simulink model "BOoe221SystReel"  (R2017a)
settings: Solver=VariableStepAuto  StartTime=0.0  StopTime=1000  RelTol=1e-9
values from neighbouring files (symbols this model uses):
  Ac75 = [26.3183614036 4.0966592869 -1.20233311116 0.735865601479 -0.745822636963 1.2499757532 -4.34795583254 -48.1646836676 11.3086114423 8.50188757288 -3.89847108842 3.46848516105 ... (49 elements, 7x7)]    [robot_75.mat]
  B = oe221.B    [main.m]
  Bc75 = [3.2987807581 -0.797878528803 0.404454582357 -0.331411019122 0.414411617841 -0.835564135359 3.51239169718]    [robot_75.mat]
  Cc75 = [0.0368 0.0059 -0.1248 0.3042 -0.2181 0.0895 0]    [robot_75.mat]
  F = oe221.F    [main.m]
  Te = 0.07    [robot_0.mat]    (also in robot_25.mat; robot_75.mat)
undefined symbols (not defined in the file or in its folder): DiscIntNeverNeededParam
libraries: simulink x2
settings Model: Creator=GANOU Arouna  LastModifiedBy=GANOU Arouna

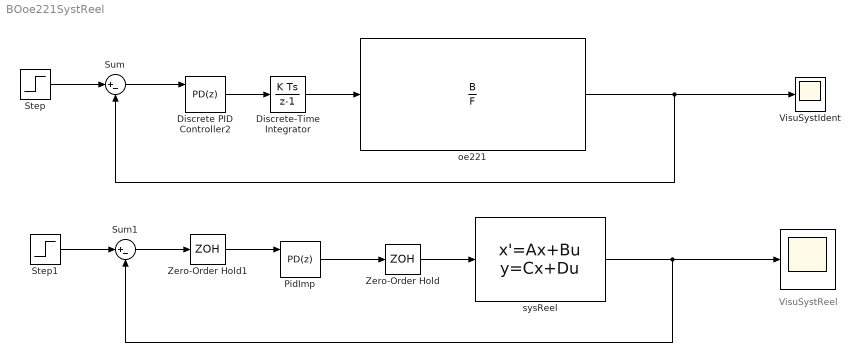
== system BOoe221SystReel ==
  note: VisuSystReel
  " " : Scope
  Discrete PID Controller2 : simulink/Continuous/PID Controller  Controller=PD  TimeDomain=Discrete-time  SampleTime=Te  IntegratorMethod=Forward Euler  FilterMethod=Forward Euler  Form=Parallel  UseFilter=on  ControllerParametersSource=internal  P=0.00429057698105191  I=0.0008007758385471  D=0  N=100  InitialConditionSource=internal  InitialConditionForIntegrator=0  InitialConditionForFilter=0  ExternalReset=either  LimitOutput=off  UpperSaturationLimit=inf  LowerSaturationLimit=-inf  LinearizeAsGain=off  AntiWindupMode=none  Kb=1  TrackingMode=off  Kt=1  PParamMin=[]  PParamMax=[]  IParamMin=[]  IParamMax=[]  DParamMin=[]  DParamMax=[]  NParamMin=[]  NParamMax=[]  KbParamMin=[]  KbParamMax=[]  KtParamMin=[]  KtParamMax=[]  POutMin=[]  POutMax=[]  IOutMin=[]  IOutMax=[]  DOutMin=[]  DOutMax=[]  NOutMin=[]  NOutMax=[]  KbOutMin=[]  KbOutMax=[]  KtOutMin=[]  KtOutMax=[]  IntegratorOutMin=[]  IntegratorOutMax=[]  FilterOutMin=[]  FilterOutMax=[]  SumOutMin=[]  SumOutMax=[]  SumI1OutMin=[]  SumI1OutMax=[]  SumI2OutMin=[]  SumI2OutMax=[]  SumI3OutMin=[]  SumI3OutMax=[]  SumDOutMin=[]  SumDOutMax=[]  SaturationOutMin=[]  SaturationOutMax=[]  IntegratorContinuousStateAttributes=''  IntegratorStateMustResolveToSignalObject=off  IntegratorRTWStateStorageClass=Auto  FilterContinuousStateAttributes=''  FilterStateMustResolveToSignalObject=off  FilterRTWStateStorageClass=Auto  DifferentiatorICPrevScaledInput=0  DifferentiatorOutMin=[]  DifferentiatorOutMax=[]  InitialConditionSetting=State (most efficient)
  Discrete-Time Integrator : DiscreteIntegrator  InitialConditionSetting=State (most efficient)  SampleTime=Te  ICPrevOutput=DiscIntNeverNeededParam  ICPrevScaledInput=DiscIntNeverNeededParam
  PidImp : simulink/Continuous/PID Controller  Controller=PD  TimeDomain=Discrete-time  SampleTime=Te  IntegratorMethod=Forward Euler  FilterMethod=Forward Euler  Form=Parallel  UseFilter=on  ControllerParametersSource=internal  P=0.00429057698105191  I=0.0008007758385471  D=0  N=100  InitialConditionSource=internal  InitialConditionForIntegrator=0  InitialConditionForFilter=0  ExternalReset=either  LimitOutput=off  UpperSaturationLimit=inf  LowerSaturationLimit=-inf  LinearizeAsGain=off  AntiWindupMode=none  Kb=1  TrackingMode=off  Kt=1  PParamMin=[]  PParamMax=[]  IParamMin=[]  IParamMax=[]  DParamMin=[]  DParamMax=[]  NParamMin=[]  NParamMax=[]  KbParamMin=[]  KbParamMax=[]  KtParamMin=[]  KtParamMax=[]  POutMin=[]  POutMax=[]  IOutMin=[]  IOutMax=[]  DOutMin=[]  DOutMax=[]  NOutMin=[]  NOutMax=[]  KbOutMin=[]  KbOutMax=[]  KtOutMin=[]  KtOutMax=[]  IntegratorOutMin=[]  IntegratorOutMax=[]  FilterOutMin=[]  FilterOutMax=[]  SumOutMin=[]  SumOutMax=[]  SumI1OutMin=[]  SumI1OutMax=[]  SumI2OutMin=[]  SumI2OutMax=[]  SumI3OutMin=[]  SumI3OutMax=[]  SumDOutMin=[]  SumDOutMax=[]  SaturationOutMin=[]  SaturationOutMax=[]  IntegratorContinuousStateAttributes=''  IntegratorStateMustResolveToSignalObject=off  IntegratorRTWStateStorageClass=Auto  FilterContinuousStateAttributes=''  FilterStateMustResolveToSignalObject=off  FilterRTWStateStorageClass=Auto  DifferentiatorICPrevScaledInput=0  DifferentiatorOutMin=[]  DifferentiatorOutMax=[]  InitialConditionSetting=State (most efficient)
  Step : Step  SampleTime=Te
  Step1 : Step  After=10  SampleTime=Te
  Sum : Sum  Inputs=|+-
  Sum1 : Sum  Inputs=|+-
  VisuSystIdent : Scope
  Zero-Order Hold : ZeroOrderHold  SampleTime=Te
  Zero-Order Hold1 : ZeroOrderHold  SampleTime=Te
  oe221 : DiscreteTransferFcn  Numerator=B  Denominator=F  SampleTime=Te
  sysReel : StateSpace  A=Ac75  B=Bc75  C=Cc75  D=0  X0=0
  wires:
  oe221/1 -> VisuSystIdent/1, Sum/2
  Step/1 -> Sum/1
  Discrete PID Controller2/1 -> Discrete-Time Integrator/1
  Discrete-Time Integrator/1 -> oe221/1
  Zero-Order Hold/1 -> sysReel/1
  Step1/1 -> Sum1/1
  sysReel/1 -> Sum1/2, " "/1
  Sum1/1 -> Zero-Order Hold1/1
  Zero-Order Hold1/1 -> PidImp/1
  PidImp/1 -> Zero-Order Hold/1
  Sum/1 -> Discrete PID Controller2/1
